simulink model "melisaaslan_adaptive_control"  (R2023b)
settings: Solver=VariableStepAuto  StartTime=0.0  StopTime=150  FixedStep=0.01  MaxStep=0.001  RelTol=1e-4
settings Model: Creator=sukrunver  LastModifiedBy=melis
settings SolverCC: AlgebraicLoopSolver=TrustRegion
settings SFSimCC: CustomCodeUndefinedFunction=UseInterfaceOnly

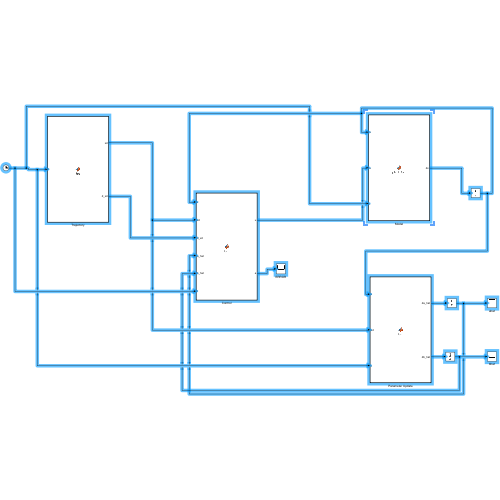
[thumbnail: Simulink's stored preview of the top-level diagram]
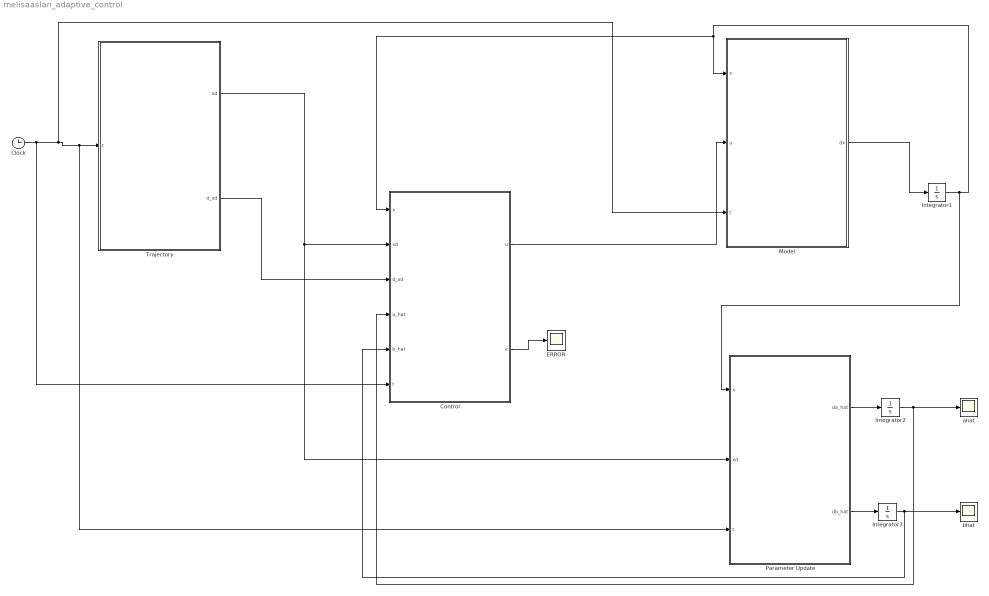
== system melisaaslan_adaptive_control ==
  Clock : Clock
  Control : MATLAB Function  TreatAsAtomicUnit=on
  ERROR : Scope
  Integrator1 : Integrator
  Integrator2 : Integrator
  Integrator3 : Integrator
  Model : MATLAB Function  TreatAsAtomicUnit=on
  Parameter Update : MATLAB Function  TreatAsAtomicUnit=on
  Trajectory : MATLAB Function  TreatAsAtomicUnit=on
  ahat : Scope
  bhat : Scope
  wires:
  Clock/1 -> Control/6(t), Model/3(t), Parameter Update/3(t), Trajectory/1(t)
  Model/1(dx) -> Integrator1/1
  Parameter Update/2(db_hat) -> Integrator3/1
  Parameter Update/1(da_hat) -> Integrator2/1
  Control/2(e) -> ERROR/1
  Control/1(u) -> Model/2(u)
  Trajectory/1(xd) -> Parameter Update/2(xd), Control/2(xd)
  Trajectory/2(d_xd) -> Control/3(d_xd)
  Integrator1/1 -> Parameter Update/1(x), Control/1(x), Model/1(x)
  Integrator2/1 -> Control/4(a_hat), ahat/1
  Integrator3/1 -> Control/5(b_hat), bhat/1

== matlab function melisaaslan_adaptive_control/Trajectory ==
  data: t input; xd output; d_xd output
function [xd, d_xd] = fcn(t)
    xd   = sin(t);
    d_xd = cos(t);

== matlab function melisaaslan_adaptive_control/Model ==
  data: x input; u input; dx output; t input
function dx = plant_fcn(x,u, t)
     a_gercek = 2.0;
     b_gercek = 1.0;
     f = a_gercek * x * cos(t) + b_gercek * sin(t);
     dx = f + u;
 end

== matlab function melisaaslan_adaptive_control/Control ==
  data: x input; xd input; d_xd input; a_hat input; b_hat input; u output; t input; e output
function [u, e] = fcn(x, xd, d_xd, a_hat, b_hat, t)
    k = 15;
    e      = xd - x;
    f_hat  = a_hat * x * cos(t) + b_hat * sin(t);
    u      = d_xd - f_hat + k * e;

== matlab function melisaaslan_adaptive_control/Parameter Update ==
  data: x input; xd input; t input; da_hat output; db_hat output
function [da_hat, db_hat] = fcn(x, xd, t)
    gamma_a = 2;
    gamma_b = 2;

    e     = xd - x;          
    phi_a = x * cos(t);
    phi_b = sin(t);

    da_hat = -gamma_a * phi_a * e;
    db_hat = -gamma_b * phi_b * e;
